simulink model "verify_HX_finned_tube_stratified_mdl"  (R2016b)
settings: Solver=VariableStepDiscrete  StartTime=0  StopTime=20  MaxStep=0.2  RelTol=1e-3  EnableMultiTasking=on
InitFcn:
  | height =1.47;
  | dia = 0.525;
  | nodes = 5;
libraries: carnot x2, simulink x1
settings Model: Creator=drhf  LastModifiedBy=drhf
settings DataIOCC: SaveFormat=Array  SignalLoggingSaveFormat=ModelDataLogs
settings OptimizationCC: ExpressionDepthLimit=2147483647  LifeSpan=inf
settings DebuggingCC: UnderspecifiedInitializationDetection=Classic  MergeDetectMultiDrivingBlocksExec=none  SolverPrmCheckMsg=warning  FcnCallInpInsideContextMsg=warning  StateNameClashWarn=warning  SFUnexpectedBacktrackingDiag=warning  SFNoUnconditionalDefaultTransitionDiag=warning  SFExecutionAtInitializationDiag=none
settings HardwareCC: ProdBitPerPointer=32  ProdBitPerSizeT=32  ProdBitPerPtrDiffT=32  ProdLargestAtomicFloat=None  ProdIntDivRoundTo=Undefined  ProdEndianess=Unspecified  ProdWordSize=32  ProdHWDeviceType=32-bit Generic
settings ModelReferenceCC: PropagateSignalLabelsOutOfModel=off
settings GRTTargetCC: TargetLangStandard=C89/C90 (ANSI)  GeneratePreprocessorConditionals=Disable all  CombineOutputUpdateFcns=off  GRTInterface=on
settings ConfigComp: CovMetricSettings=dw  CovHtmlReporting=on  CovSaveCumulativeToWorkspaceVar=on  CovSaveSingleToWorkspaceVar=on  CovExternalEMLEnable=off

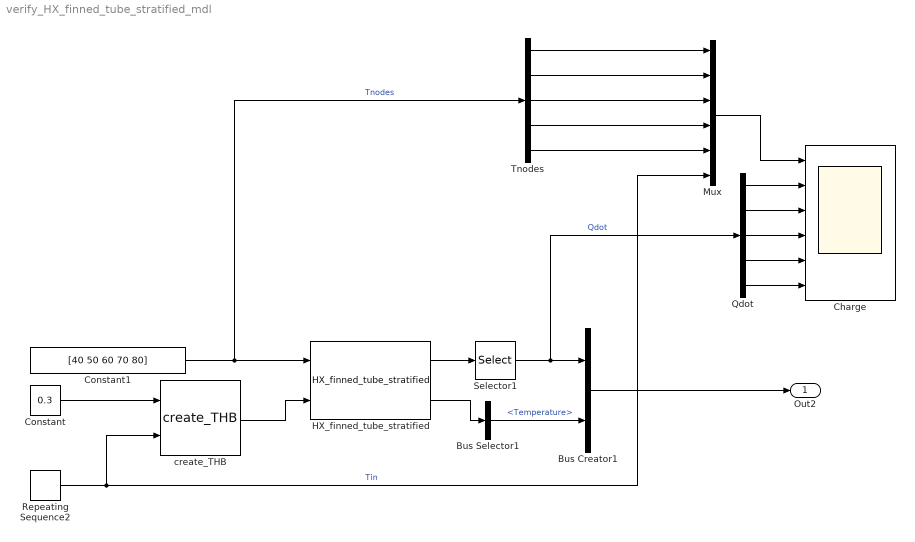
== system verify_HX_finned_tube_stratified_mdl ==
  Bus Creator1 : BusCreator  Inputs=2
  Bus Selector1 : BusSelector  OutputSignals=Temperature
  Charge : Scope  NumInputPorts=6
  Constant : Constant  Value=0.3
  Constant1 : Constant  Value=[40 50 60 70 80]
  HX_finned_tube_stratified : carnot/Storage/Thermal/Storage_Ports/HX_finned_tube_stratified  h_in=0.9  h_out=0.1  hgt=1  dpipe=0.03  swall=0.002  lpipe=15  cond=50  dfin=0.05  sfin=0.001  nfin=100  height=-0.8  dplin=100  dpqua=100  nodes=5
  Mux : Mux  Inputs=6
  Qdot : Demux  Outputs=5
  Repeating Sequence2 : simulink/Sources/Repeating Sequence  rep_seq_t=[0 5 10]  rep_seq_y=[30 90 30]
  Selector1 : Selector  InputPortWidth=28  IndexOptions=Index vector (dialog)  Indices=[21:25]  OutputSizes=1
  Tnodes : Demux  Outputs=5
  create_THB : carnot/Source/Simple/create_THB  p=1e5  fluid=Water  mix=0  mix2=0  mix3=0  dia=0.02  hgt=0  mID=No Pressure Drop
  Out2 : Outport
  wires:
  HX_finned_tube_stratified/1 -> Selector1/1
  HX_finned_tube_stratified/2 -> Bus Selector1/1
  Selector1/1 -> Qdot/1, Bus Creator1/1  "Qdot"
  Bus Selector1/1 -> Bus Creator1/2  "<Temperature>"
  Bus Creator1/1 -> Out2/1
  Constant1/1 -> Tnodes/1, HX_finned_tube_stratified/1  "Tnodes"
  create_THB/1 -> HX_finned_tube_stratified/2
  Constant/1 -> create_THB/1
  Repeating Sequence2/1 -> create_THB/2, Mux/6  "Tin"
  Mux/1 -> Charge/1
  Qdot/3 -> Charge/4
  Qdot/2 -> Charge/3
  Qdot/4 -> Charge/5
  Qdot/5 -> Charge/6
  Qdot/1 -> Charge/2
  Tnodes/4 -> Mux/4
  Tnodes/1 -> Mux/1
  Tnodes/3 -> Mux/3
  Tnodes/2 -> Mux/2
  Tnodes/5 -> Mux/5
